simulink model "Encryption_App"  (R2023a)
settings: Solver=FixedStepAuto  StartTime=0.0  StopTime=10.0  RelTol=1e-3
libraries: androiduilib x2, dspsrcs4 x2, androidaudiovideolib x1, androidcommunicationlib x1
settings Model: Creator=ragha  LastModifiedBy=ragha
settings OptimizationCC: EnhancedBackFolding=on  PassReuseOutputArgsAs=Individual arguments  ZeroExternalMemoryAtStartup=off  ZeroInternalMemoryAtStartup=off  MaxStackSize=64  OptimizeBlockOrder=speed  DifferentSizesBufferReuse=on  OptimizationCustomize=off  EfficientTunableParamExpr=on
settings DebuggingCC: ParameterTunabilityLossMsg=error
settings HardwareCC: ProdBitPerPointer=32  ProdBitPerSizeT=32  ProdBitPerPtrDiffT=32  ProdLargestAtomicInteger=Long  ProdLargestAtomicFloat=Double  ProdWordSize=32  ProdHWDeviceType=ARM Compatible->ARM Cortex
settings SFSimCC: MATLABDynamicMemAlloc=off
settings RTWCC: Description=Embedded Coder  SystemTargetFile=ert.tlc  HardwareBoard=Android Device  TLCOptions="-aInlineSetEventsForThisBaseRateFcn=TLC_FALSE -aSuppressMultiTaskScheduler=TLC_FALSE  -aRateBasedStepFcn=0"  TemplateMakefile=ert_default_tmf  RTWVerbose=off  Toolchain=Android SDK/NDK Tools
settings CodeAppCC: ForceParamTrailComments=on  IgnoreCustomStorageClasses=off  OperatorAnnotations=on  SimulinkDataObjDesc=on  SFDataObjDesc=on  InsertBlockDesc=on

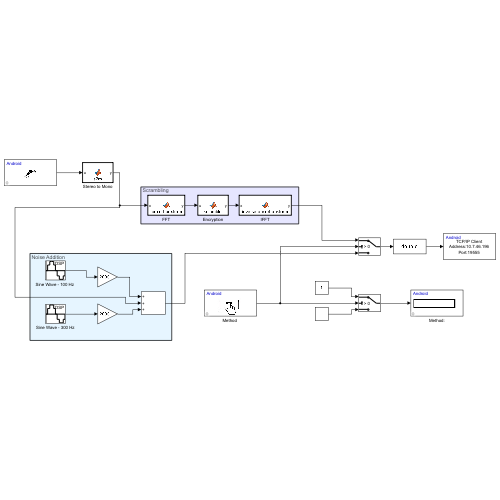
[thumbnail: Simulink's stored preview of the top-level diagram]
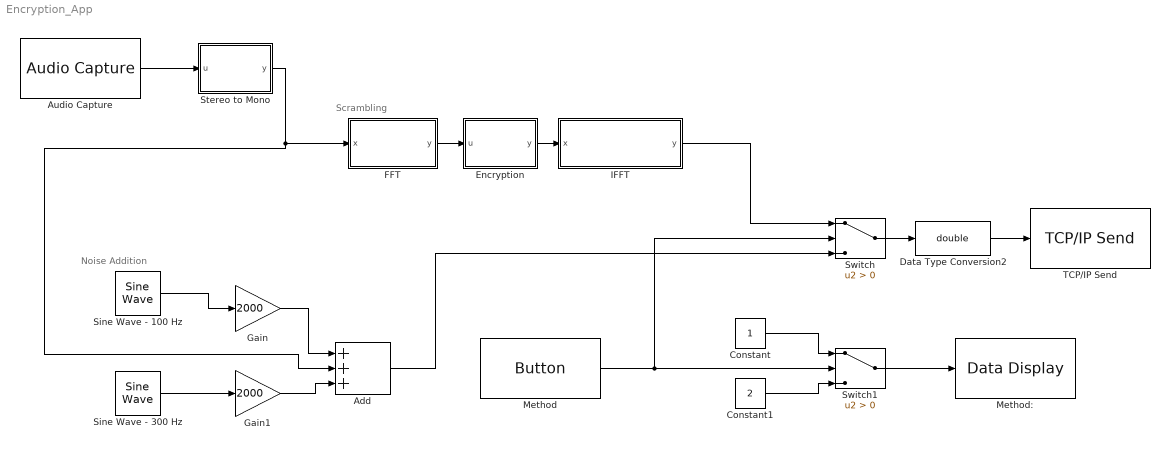
== system Encryption_App ==
  note: Noise Addition
  note: Scrambling
  Add : Sum  Inputs=+++
  Audio Capture : androidaudiovideolib/Audio Capture  SampleFreq=44100  FrameSize=441  SampleTime=0.01  SimulateUsing=Code generation  DeviceStr=0  QueueDuration=0  BlockPlatform=Android  AudioSamplingFreq=44100
  Constant : Constant
  Constant1 : Constant  Value=2
  Data Type Conversion2 : DataTypeConversion  OutDataTypeStr=double  SaturateOnIntegerOverflow=off  RndMeth=Floor
  Encryption : MATLAB Function  TreatAsAtomicUnit=on
  FFT : MATLAB Function  TreatAsAtomicUnit=on
  Gain : Gain  Gain=2000
  Gain1 : Gain  Gain=2000
  IFFT : MATLAB Function  TreatAsAtomicUnit=on
  "Method " : androiduilib/Button  ButtonState=Not pressed  ButtonId=Encryption_App/Method_  State=off  SampleTime=0.1  BlockPlatform=Android
  Method: : androiduilib/Data Display  DataDisplayId=Encryption_App/Method:  Format=Float  Precision=6  SimulateUsing=Code generation  blockPlatform=Android
  "Sine Wave - 100 Hz " : dspsrcs4/Sine Wave  Amplitude=1  Frequency=100  Phase=0  SampleMode=Discrete  OutComplex=Real  CompMethod=Trigonometric fcn  TableSize=Speed  SampleTime=1/1000  SamplesPerFrame=1  ResetState=Restart at time zero  OutputFrames=off  dataType=double  wordLen=16  udDataType=sfix(16)  fracBitsMode=Best precision  numFracBits=15  OutDataTypeStr=double  LastOutDataTypeStr=double
  Sine Wave - 300 Hz : dspsrcs4/Sine Wave  Amplitude=1  Frequency=300  Phase=0  SampleMode=Discrete  OutComplex=Real  CompMethod=Trigonometric fcn  TableSize=Speed  SampleTime=1/1000  SamplesPerFrame=1  ResetState=Restart at time zero  OutputFrames=off  dataType=double  wordLen=16  udDataType=sfix(16)  fracBitsMode=Best precision  numFracBits=15  OutDataTypeStr=double  LastOutDataTypeStr=double
  Stereo to Mono : MATLAB Function  TreatAsAtomicUnit=on
  Switch : Switch  Criteria=u2 > Threshold  SaturateOnIntegerOverflow=off  InputSameDT=off
  Switch1 : Switch  Criteria=u2 > Threshold  SaturateOnIntegerOverflow=off  InputSameDT=off
  TCP/IP Send : androidcommunicationlib/TCP//IP Send  TCPSendId=Encryption_App/TCP//IP_Send  Mode_=Client  LocalServerPort_=25000  RemoteAddr_=10.7.46.196  RemoteServerPort_=19555  ClientPortBindingSelection_=on  ClientPortToBind_=35000  BlockingMode_=off  BlockTimeout_=0.1
  wires:
  FFT/1(y) -> Encryption/1(u)
  Audio Capture/1 -> Stereo to Mono/1(u)
  Encryption/1(y) -> IFFT/1(x)
  Data Type Conversion2/1 -> TCP/IP Send/1
  "Method "/1 -> Switch/2, Switch1/2
  IFFT/1(y) -> Switch/1
  Add/1 -> Switch/3
  Switch/1 -> Data Type Conversion2/1
  Constant/1 -> Switch1/1
  Switch1/1 -> Method:/1
  Constant1/1 -> Switch1/3
  Stereo to Mono/1(y) -> Add/2, FFT/1(x)
  "Sine Wave - 100 Hz "/1 -> Gain/1
  Sine Wave - 300 Hz/1 -> Gain1/1
  Gain/1 -> Add/1
  Gain1/1 -> Add/3

== matlab function Encryption_App/FFT ==
  data: x input; y output
function y = fouriertransform(x)
    y = fft(x);
end

== matlab function Encryption_App/Encryption ==
  data: u input; y output
function y = scramble(u)

y = u*6;

== matlab function Encryption_App/Stereo to Mono ==
  data: u input; y output
function y = s2m(u)

y = u(:,1);

== matlab function Encryption_App/IFFT ==
  data: x input; y output
function y = inversefouriertransform(x)
    y = real(ifft(x));
end
